simulink model "simulation_4_10"  (R2018b)
settings: Solver=VariableStepAuto  StartTime=0.0  StopTime=10.0  RelTol=1e-3
values from neighbouring files (symbols this model uses):
  beta = 0.000001    (= 1e-06)    [params.m]    (also in params_4_10.m = 0.2)
  k = 2    [params_4_10.m]
  m = 10    [params_4_10.m]
settings Model: Creator=cale  LastModifiedBy=cale

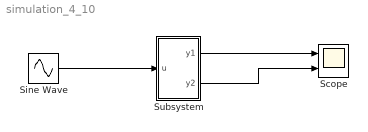
== system simulation_4_10 ==
  Scope : Scope  NumInputPorts=2
  Sine Wave : Sin  Amplitude=5  Bias=10.5  Frequency=2  SampleTime=0
  Subsystem : Subsystem
  wires:
  Sine Wave/1 -> Subsystem/1(u)
  Subsystem/1("y1 ") -> Scope/1
  Subsystem/2(y2) -> Scope/2

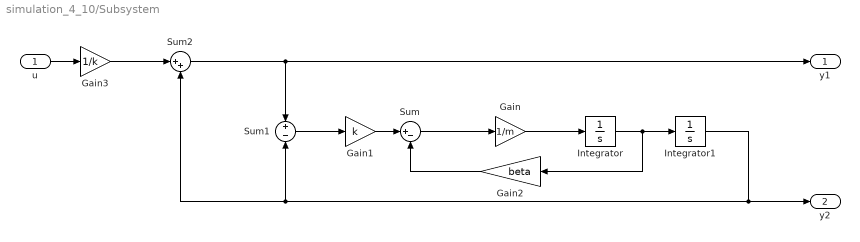
== system simulation_4_10/Subsystem ==
  u : Inport
  Gain : Gain  Gain=1/m
  Gain1 : Gain  Gain=k
  Gain2 : Gain  Gain=beta
  Gain3 : Gain  Gain=1/k
  Integrator : Integrator
  Integrator1 : Integrator
  Sum : Sum  Inputs=|+-
  Sum1 : Sum  Inputs=+|-
  Sum2 : Sum  Inputs=|++
  "y1 " : Outport
  y2 : Outport  Port=2
  wires:
  Integrator/1 -> Gain2/1, Integrator1/1
  Sum/1 -> Gain/1
  Gain/1 -> Integrator/1
  Sum1/1 -> Gain1/1
  Gain1/1 -> Sum/1
  Integrator1/1 -> Sum2/2, Sum1/2, y2/1
  Gain2/1 -> Sum/2
  Sum2/1 -> Sum1/1, "y1 "/1
  u/1 -> Gain3/1
  Gain3/1 -> Sum2/1
